simulink model "MSP_CurrentControl"  (R2018a)
settings: Solver=ode15s  StartTime=0.0  StopTime=1  RelTol=1e-3
values from neighbouring files (symbols this model uses):
  Kd = 0    [init.m]
  Ki = 63    [init.m]
  Kp = 6.3    [init.m]
  L = 1e-1    (= 0.1)    [init.m]
  n_levels = 9    [init.m]
  R = 90    [init.m]
  reference_frequency_hz = 100    [init.m]
  Ts = 1e-4    (= 0.0001)    [init.m]
  Vdc = 1    [init.m]
undefined symbols (not defined in the file or in its folder): G, serial
libraries: elec_lib x63, nesl_utility x52, powerlib x41, fl_lib x40, powerlib_meascontrol x4, simulink x3, instrumentlib x3
(part 1 of 2)
settings Model: Creator=Lewis  LastModifiedBy=Lewis
settings SolverCC: AutoInsertRateTranBlk=on  InsertRTBMode=Never (minimum delay)
settings SimscapeCC: SimscapeLogType=all

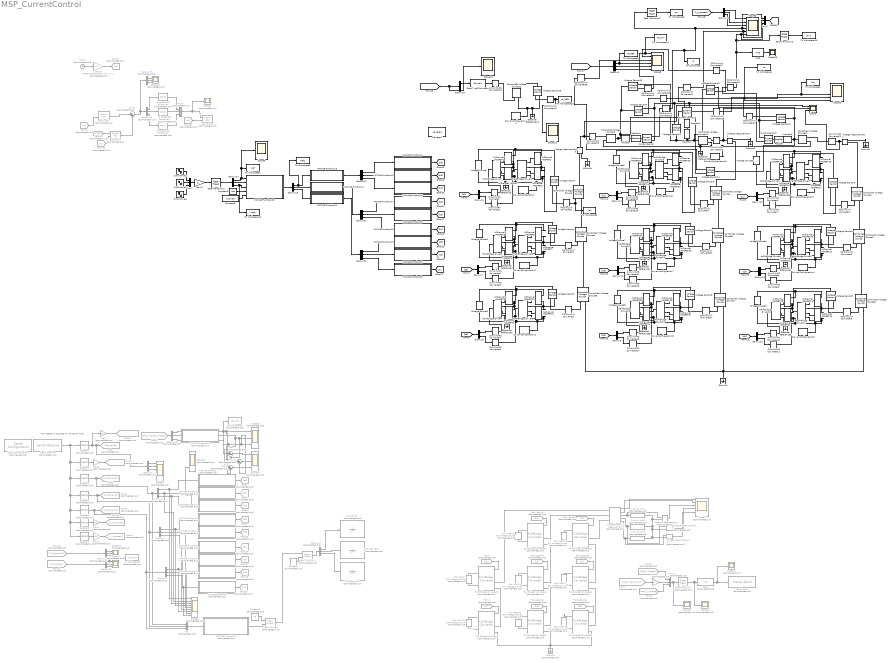
== system MSP_CurrentControl ==
  note: The header is dropped by the serial block
  1 ohm 5 mH1 : powerlib/Elements/Series RLC Branch  Commented=on  LConnTagsString=__new0  RConnTagsString=__new0  BranchType=RL  Resistance=R  Inductance=L  SetiL0=off  InitialCurrent=0  Capacitance=400e-6  Setx0=off  InitialVoltage=0  Measurements=None
  1 ohm 5 mH2 : powerlib/Elements/Series RLC Branch  Commented=on  LConnTagsString=__new0  RConnTagsString=__new0  BranchType=RL  Resistance=R  Inductance=L  SetiL0=off  InitialCurrent=0  Capacitance=400e-6  Setx0=off  InitialVoltage=0  Measurements=None
  1 ohm 5 mH3 : powerlib/Elements/Series RLC Branch  Commented=on  LConnTagsString=__new0  RConnTagsString=__new0  BranchType=RL  Resistance=R  Inductance=L  SetiL0=on  InitialCurrent=0  Capacitance=400e-6  Setx0=off  InitialVoltage=0  Measurements=None
  Cast : DataTypeConversion  Commented=on  OutDataTypeStr=int8  SaturateOnIntegerOverflow=on
  Clock1 : Clock  Commented=on
  Constant : Constant  Commented=on  Value=[9;3;1]
  Constant1 : Constant  Commented=on  Value=G
  Constant2 : Constant  Value=Vdc
  Constant3 : Constant  Value=n_levels
  Controlled Voltage Source{9..12} (4 alike) : fl_lib/Electrical/Electrical Sources/Controlled Voltage Source
  Controlled Voltage Source{,1..8} (9 alike) : powerlib/Electrical Sources/Controlled Voltage Source  Initialize=on  Source_Type=AC  Amplitude=0  Phase=0  Frequency=0  Measurements=None
  Current Sensor : fl_lib/Electrical/Electrical Sensors/Current Sensor
  Current Sensor1 : fl_lib/Electrical/Electrical Sensors/Current Sensor
  Current Sensor2 : fl_lib/Electrical/Electrical Sensors/Current Sensor
  Data Type Conversion : DataTypeConversion
  Demux{1..4,14..15,17..19,25} (10 alike) : Demux  Commented=on  Outputs=3
  Demux{6..13,16} (9 alike) : Demux  Outputs=2
  Demux{5,20..24,26..27} (8 alike) : Demux  Outputs=3
  Discrete PID Controller : simulink/Continuous/PID Controller  Commented=on  Controller=PID  TimeDomain=Discrete-time  SampleTime=-1  IntegratorMethod=Forward Euler  FilterMethod=Forward Euler  Form=Parallel  UseFilter=on  ControllerParametersSource=internal  P=Kp  I=Ki  D=Kd  N=100  InitialConditionSource=internal  InitialConditionForIntegrator=0  InitialConditionForFilter=0  ExternalReset=none  LimitOutput=off  UpperSaturationLimit=inf  LowerSaturationLimit=-inf  LinearizeAsGain=off  AntiWindupMode=none  Kb=1  TrackingMode=off  Kt=1  PParamMin=[]  PParamMax=[]  IParamMin=[]  IParamMax=[]  DParamMin=[]  DParamMax=[]  NParamMin=[]  NParamMax=[]  KbParamMin=[]  KbParamMax=[]  KtParamMin=[]  KtParamMax=[]  POutMin=[]  POutMax=[]  IOutMin=[]  IOutMax=[]  DOutMin=[]  DOutMax=[]  NOutMin=[]  NOutMax=[]  KbOutMin=[]  KbOutMax=[]  KtOutMin=[]  KtOutMax=[]  IntegratorOutMin=[]  IntegratorOutMax=[]  FilterOutMin=[]  FilterOutMax=[]  SumOutMin=[]  SumOutMax=[]  SumI1OutMin=[]  SumI1OutMax=[]  SumI2OutMin=[]  SumI2OutMax=[]  SumI3OutMin=[]  SumI3OutMax=[]  SumDOutMin=[]  SumDOutMax=[]  SaturationOutMin=[]  SaturationOutMax=[]  IntegratorContinuousStateAttributes=''  IntegratorStateMustResolveToSignalObject=off  IntegratorRTWStateStorageClass=Auto  FilterContinuousStateAttributes=''  FilterStateMustResolveToSignalObject=off  FilterRTWStateStorageClass=Auto  DifferentiatorICPrevScaledInput=0  DifferentiatorOutMin=[]  DifferentiatorOutMax=[]  FilterDiffOutCoefMin=[]  FilterDiffOutCoefMax=[]  SumDenOutMin=[]  SumDenOutMax=[]  SumNumOutMin=[]  SumNumOutMax=[]  ReciprocalOutMin=[]  ReciprocalOutMax=[]  DivideOutMin=[]  DivideOutMax=[]  TunerSelectOption=Transfer Function Based (PID Tuner App)
  Discrete PID Controller1 : simulink/Continuous/PID Controller  Commented=on  Controller=PID  TimeDomain=Discrete-time  SampleTime=-1  IntegratorMethod=Forward Euler  FilterMethod=Forward Euler  Form=Parallel  UseFilter=on  ControllerParametersSource=internal  P=Kp  I=Ki  D=Kd  N=100  InitialConditionSource=internal  InitialConditionForIntegrator=0  InitialConditionForFilter=0  ExternalReset=none  LimitOutput=off  UpperSaturationLimit=inf  LowerSaturationLimit=-inf  LinearizeAsGain=off  AntiWindupMode=none  Kb=1  TrackingMode=off  Kt=1  PParamMin=[]  PParamMax=[]  IParamMin=[]  IParamMax=[]  DParamMin=[]  DParamMax=[]  NParamMin=[]  NParamMax=[]  KbParamMin=[]  KbParamMax=[]  KtParamMin=[]  KtParamMax=[]  POutMin=[]  POutMax=[]  IOutMin=[]  IOutMax=[]  DOutMin=[]  DOutMax=[]  NOutMin=[]  NOutMax=[]  KbOutMin=[]  KbOutMax=[]  KtOutMin=[]  KtOutMax=[]  IntegratorOutMin=[]  IntegratorOutMax=[]  FilterOutMin=[]  FilterOutMax=[]  SumOutMin=[]  SumOutMax=[]  SumI1OutMin=[]  SumI1OutMax=[]  SumI2OutMin=[]  SumI2OutMax=[]  SumI3OutMin=[]  SumI3OutMax=[]  SumDOutMin=[]  SumDOutMax=[]  SaturationOutMin=[]  SaturationOutMax=[]  IntegratorContinuousStateAttributes=''  IntegratorStateMustResolveToSignalObject=off  IntegratorRTWStateStorageClass=Auto  FilterContinuousStateAttributes=''  FilterStateMustResolveToSignalObject=off  FilterRTWStateStorageClass=Auto  DifferentiatorICPrevScaledInput=0  DifferentiatorOutMin=[]  DifferentiatorOutMax=[]  FilterDiffOutCoefMin=[]  FilterDiffOutCoefMax=[]  SumDenOutMin=[]  SumDenOutMax=[]  SumNumOutMin=[]  SumNumOutMax=[]  ReciprocalOutMin=[]  ReciprocalOutMax=[]  DivideOutMin=[]  DivideOutMax=[]  TunerSelectOption=Transfer Function Based (PID Tuner App)
  Discrete PID Controller2 : simulink/Continuous/PID Controller  Commented=on  Controller=PID  TimeDomain=Discrete-time  SampleTime=-1  IntegratorMethod=Forward Euler  FilterMethod=Forward Euler  Form=Parallel  UseFilter=on  ControllerParametersSource=internal  P=Kp  I=Ki  D=Kd  N=100  InitialConditionSource=internal  InitialConditionForIntegrator=0  InitialConditionForFilter=0  ExternalReset=none  LimitOutput=off  UpperSaturationLimit=inf  LowerSaturationLimit=-inf  LinearizeAsGain=off  AntiWindupMode=none  Kb=1  TrackingMode=off  Kt=1  PParamMin=[]  PParamMax=[]  IParamMin=[]  IParamMax=[]  DParamMin=[]  DParamMax=[]  NParamMin=[]  NParamMax=[]  KbParamMin=[]  KbParamMax=[]  KtParamMin=[]  KtParamMax=[]  POutMin=[]  POutMax=[]  IOutMin=[]  IOutMax=[]  DOutMin=[]  DOutMax=[]  NOutMin=[]  NOutMax=[]  KbOutMin=[]  KbOutMax=[]  KtOutMin=[]  KtOutMax=[]  IntegratorOutMin=[]  IntegratorOutMax=[]  FilterOutMin=[]  FilterOutMax=[]  SumOutMin=[]  SumOutMax=[]  SumI1OutMin=[]  SumI1OutMax=[]  SumI2OutMin=[]  SumI2OutMax=[]  SumI3OutMin=[]  SumI3OutMax=[]  SumDOutMin=[]  SumDOutMax=[]  SaturationOutMin=[]  SaturationOutMax=[]  IntegratorContinuousStateAttributes=''  IntegratorStateMustResolveToSignalObject=off  IntegratorRTWStateStorageClass=Auto  FilterContinuousStateAttributes=''  FilterStateMustResolveToSignalObject=off  FilterRTWStateStorageClass=Auto  DifferentiatorICPrevScaledInput=0  DifferentiatorOutMin=[]  DifferentiatorOutMax=[]  FilterDiffOutCoefMin=[]  FilterDiffOutCoefMax=[]  SumDenOutMin=[]  SumDenOutMax=[]  SumNumOutMin=[]  SumNumOutMax=[]  ReciprocalOutMin=[]  ReciprocalOutMax=[]  DivideOutMin=[]  DivideOutMax=[]  TunerSelectOption=Transfer Function Based (PID Tuner App)
  Electrical Reference{,1..10} (11 alike) : fl_lib/Electrical/Electrical Elements/Electrical Reference
  From : From  Commented=on  GotoTag=a3
  From1 : From  Commented=on  GotoTag=a9
  From10 : From  Commented=on  GotoTag=V_XN_sensed
  From11 : From  Commented=on  GotoTag=I_ll_sensed
  From2 : From  Commented=on  GotoTag=abc_inverter_voltage
  From20 : From  Commented=on  GotoTag=I_meas
  From21 : From  Commented=on  GotoTag=wt
  From22 : From  Commented=on  GotoTag=wt
  From23 : From  Commented=on  GotoTag=wt
  From3 : From  Commented=on  GotoTag=load_voltage
  From4 : From  Commented=on  GotoTag=load_line_current
  From5 : From  Commented=on  GotoTag=load_ll_voltage
  From_Boost1 : From  Commented=on  GotoTag=b1
  From_Boost2 : From  Commented=on  GotoTag=c1
  From_Boost3 : From  Commented=on  GotoTag=c3
  From_Boost4 : From  Commented=on  GotoTag=c9
  From_Boost5 : From  Commented=on  GotoTag=b3
  From_Boost6 : From  Commented=on  GotoTag=b9
  Full-Bridge Converter : powerlib/Power Electronics/Full-Bridge Converter  Commented=on  ModelType=Switching devices  Ron=Ron  Rs=1e6  Cs=1e-3  Vforward=[ 0, 0 ]  Ron_Diode=1e-3  Rs_Diode=1e6  Cs_Diode=inf  Vf_Diode=1e-3  Rs_CurrentSource=1
      settings: AttributesFormatString=%<ModelType>  SourceProductName=Simscape Power Systems  SourceProductBaseCode=PS
  Full-Bridge Converter{1,4..8} (6 alike) : powerlib/Power Electronics/Full-Bridge Converter  Commented=on  ModelType=Switching devices  Ron=Ron  Rs=1e6  Cs=inf  Vforward=[ 0, 0 ]  Ron_Diode=1e-3  Rs_Diode=1e6  Cs_Diode=inf  Vf_Diode=1e-3  Rs_CurrentSource=1
      settings: AttributesFormatString=%<ModelType>  SourceProductName=Simscape Power Systems  SourceProductBaseCode=PS
  Full-Bridge Converter2 : powerlib/Power Electronics/Full-Bridge Converter  Commented=on  ModelType=Switching devices  Ron=Ron  Rs=1e6  Cs=1e-3  Vforward=[ 0, 0 ]  Ron_Diode=1e-3  Rs_Diode=1e6  Cs_Diode=inf  Vf_Diode=1e-3  Rs_CurrentSource=1
      settings: AttributesFormatString=%<ModelType>  SourceProductName=Simscape Power Systems  SourceProductBaseCode=PS
  Gain : Gain  Commented=on  Gain=Vdc
  Gain2 : Gain  Commented=on  Gain=64
  Gain3 : Gain  Commented=on  Gain=1/20
  Gain4 : Gain  Commented=on  Gain=1/2
  Gain5 : Gain  Gain=6
  Gain6 : Gain  Commented=on  Gain=reference_frequency_hz * 2 * pi
  Gain7 : Gain  Commented=on  Gain=1/64
  Goto : Goto  Commented=on  GotoTag=abc_levels
  Goto1 : Goto  Commented=on  GotoTag=ll_abc_reference
  Goto10 : Goto  Commented=on  GotoTag=V_XN_sensed
  Goto11 : Goto  Commented=on  GotoTag=I_ll_sensed
  Goto12 : Goto  Commented=on  GotoTag=b3
  Goto13 : Goto  Commented=on  GotoTag=b1
  Goto14 : Goto  Commented=on  GotoTag=c9
  Goto15 : Goto  Commented=on  GotoTag=c3
  Goto16 : Goto  Commented=on  GotoTag=c1
  Goto2 : Goto  Commented=on  GotoTag=a9
  Goto27 : Goto  Commented=on  GotoTag=wt
  Goto3 : Goto  Commented=on  GotoTag=a_cell_levels
  Goto4 : Goto  Commented=on  GotoTag=b_cell_levels
  Goto5 : Goto  Commented=on  GotoTag=c_cell_levels
  Goto6 : Goto  Commented=on  GotoTag=abc_inverter_voltage
  Goto7 : Goto  Commented=on  GotoTag=a3
  Goto8 : Goto  Commented=on  GotoTag=a1
  Goto9 : Goto  Commented=on  GotoTag=b9
  Ground : powerlib/Elements/Ground  Commented=on  LConnTagsString=a
  Ground{1..4} (4 alike) : powerlib/Elements/Ground  LConnTagsString=a
  Half-Bridge Driver{,1..17} (18 alike) : elec_lib/Actuators & Drivers/Drivers/Half-Bridge Driver  vHigh=15 V  vLow=0 V  parameterization=1  rHigh=2 Ohm  rLow=2 Ohm  tRise=20 ns  tFall=20 ns  cLoad=10 nF  enable_faults=0  t_fault=1 s  fault_type=1  uHighValue=0.7  uLowValue=0.3  tpLH=50 ns  tdLH=100 ns  tpHL=50 ns  tdHL=100 ns  ZonTime_specify=off  ZonTime_priority=None  ZonTime=0 s  ZoffTime_specify=off  ZoffTime_priority=None  ZoffTime=0 s  power_dissipated_high_side_specify=off  power_dissipated_high_side_priority=None  power_dissipated_high_side=0 W  power_dissipated_high_side_nominal_specify=off  power_dissipated_high_side_nominal_unit=W  power_dissipated_high_side_nominal_value=1  power_dissipated_low_side_specify=off  power_dissipated_low_side_priority=None  power_dissipated_low_side=0 W  power_dissipated_low_side_nominal_specify=off  power_dissipated_low_side_nominal_unit=W  power_dissipated_low_side_nominal_value=1  uHigh=2.0 V  uLow=0.8 V
      settings: SourceProductName=Simscape Electronics  SourceProductBaseCode=SN
  Inductor : fl_lib/Electrical/Electrical Elements/Inductor  l=L H  r=0 Ohm  g=1e-9 1/Ohm  i_specify=off  i_priority=None  i=0 A  i_nominal_specify=off  i_nominal_unit=A  i_nominal_value=1  v_specify=off  v_priority=None  v=0 V  v_nominal_specify=off  v_nominal_unit=V  v_nominal_value=1  i_L_specify=off  i_L_priority=High  i_L=0 A  i_L_nominal_specify=off  i_L_nominal_unit=A  i_L_nominal_value=1
  Inductor1 : fl_lib/Electrical/Electrical Elements/Inductor  l=L H  r=0 Ohm  g=1e-9 1/Ohm  i_specify=off  i_priority=None  i=0 A  i_nominal_specify=off  i_nominal_unit=A  i_nominal_value=1  v_specify=off  v_priority=None  v=0 V  v_nominal_specify=off  v_nominal_unit=V  v_nominal_value=1  i_L_specify=off  i_L_priority=High  i_L=0 A  i_L_nominal_specify=off  i_L_nominal_unit=A  i_L_nominal_value=1
  Inductor2 : fl_lib/Electrical/Electrical Elements/Inductor  l=L H  r=0 Ohm  g=1e-9 1/Ohm  i_specify=off  i_priority=None  i=0 A  i_nominal_specify=off  i_nominal_unit=A  i_nominal_value=1  v_specify=off  v_priority=None  v=0 V  v_nominal_specify=off  v_nominal_unit=V  v_nominal_value=1  i_L_specify=off  i_L_priority=High  i_L=0 A  i_L_nominal_specify=off  i_L_nominal_unit=A  i_L_nominal_value=1
  MATLAB Function : MATLAB Function  Commented=on  TreatAsAtomicUnit=on
  MATLAB Function1 : MATLAB Function  Commented=on  TreatAsAtomicUnit=on
  MATLAB Function10 : MATLAB Function  Commented=on  TreatAsAtomicUnit=on
  MATLAB Function11 : MATLAB Function  TreatAsAtomicUnit=on
  MATLAB Function12 : MATLAB Function  TreatAsAtomicUnit=on
  MATLAB Function13 : MATLAB Function  TreatAsAtomicUnit=on
  MATLAB Function14 : MATLAB Function  TreatAsAtomicUnit=on
  MATLAB Function15 : MATLAB Function  TreatAsAtomicUnit=on
  MATLAB Function16 : MATLAB Function  TreatAsAtomicUnit=on
  MATLAB Function17 : MATLAB Function  TreatAsAtomicUnit=on
  MATLAB Function18 : MATLAB Function  TreatAsAtomicUnit=on
  MATLAB Function19 : MATLAB Function  TreatAsAtomicUnit=on
  MATLAB Function2 : MATLAB Function  Commented=on  TreatAsAtomicUnit=on
  MATLAB Function20 : MATLAB Function  TreatAsAtomicUnit=on
  MATLAB Function21 : MATLAB Function  TreatAsAtomicUnit=on
  MATLAB Function22 : MATLAB Function  TreatAsAtomicUnit=on
  MATLAB Function23 : MATLAB Function  TreatAsAtomicUnit=on
  MATLAB Function24 : MATLAB Function  Commented=on  TreatAsAtomicUnit=on
  MATLAB Function3 : MATLAB Function  Commented=on  TreatAsAtomicUnit=on
  MATLAB Function4 : MATLAB Function  Commented=on  TreatAsAtomicUnit=on
  MATLAB Function5 : MATLAB Function  Commented=on  TreatAsAtomicUnit=on
  MATLAB Function6 : MATLAB Function  Commented=on  TreatAsAtomicUnit=on
  MATLAB Function7 : MATLAB Function  Commented=on  TreatAsAtomicUnit=on
  MATLAB Function8 : MATLAB Function  Commented=on  TreatAsAtomicUnit=on
  Matrix Multiply : Product  Commented=on  Multiplication=Matrix(*)
  Matrix Multiply1 : Product  Commented=on  Multiplication=Matrix(*)
  Mux : Mux  Commented=on  Inputs=3
  Mux1 : Mux  Inputs=3
  Mux2 : Mux  Inputs=3
  Mux3 : Mux  Commented=on  Inputs=3
  Mux4 : Mux  Commented=on  Inputs=3
  N-Channel MOSFET{,4,8,12,18,22,24,30,34} (9 alike) : elec_lib/Semiconductor Devices/N-Channel MOSFET  parameterization=1  prmDatasheet=1  prmEquCoeff=1  Beta=5 A/V^2  Rds=0.025 Ohm  Id=6 A  Vgs=10 V  Vth=1.7 V  lam=0 1/V  Tmeas=25 degC  RS=1e-4 Ohm  RD=0.01 Ohm  C_param=3  C_GS=270 pF  C_GD=80 pF  C_DS=0 pF  C_iss=350 pF  C_rss=80 pF  C_oss=0 pF  C_GS_vec=[ 270 300 290 280 295 255 ] pF  C_GD_vec=[ 450 400 300 190 95 55 ] pF  C_DS_vec=[ 450 410 390 230 175 115 ] pF  C_iss_vec=[ 720 700 590 470 390 310 ] pF  C_rss_vec=[ 450 400 300 190 95 55 ] pF  C_oss_vec=[ 900 810 690 420 270 170 ] pF  C_Vds_vec=[ 0.1 0.3 1 3 10 30 ] V  V_GS_for_cap_data=0 V  charge_linearity_param=1  C_OX=200 pF  V_C_OX=-0.5 V  IsDiode=0 A  Vbi=0.6 V  n=1  Cj0Diode=0 pF  TT=50e-9 s  dVth_dT=-6 mV/K  Rds_T2=0.037 Ohm  Tmeas2=125 degC  BEXDatasheet=-1.5  BEXEquCoeff=-1.5  etaisDatasheet=3  etaisEquCoeff=3  TdeviceDatasheet=25 degC  TdeviceEquCoeff=25 degC  Rth=[1, 10] K/W  thermal_mass_parameterization=1  thermal_mass=[1, 1] J/K  thermal_time_constant=[1, 10] s  thermal_mass_initial_temperatures=[ 25 25 ] degC  betaref=18 A/V^2  Vfbref=-1.1 V  gamma=3.5 V^0.50000  phib2ref=1 V  thesatref=0.4 1/V  alpha=0  Vp=5e-2 V  thesrref=0 1/V  m=8  Tref=25 degC  Cox=1500 pF  Cgso=100 pF  Cgdo=14 pF  Rsref=2e-3 Ohm  Rdref=0.17 Ohm  Rgref=8.4 Ohm  Isref=5.2e-13 A  Cj0=480 pF  Tprm=1  etabet=1.3  Stvfb=5e-4 V/K  Stphib=-8.5e-4 V/K  etasat=1.04  etasr=0.65  etar=0.95  etais=3  Tsim=25 degC  T0=[25, 25] degC
      settings: SourceProductName=Simscape Electronics  SourceProductBaseCode=SN
  N-Channel MOSFET{1..3,5..7,9..11,13..17,19..21,23,26..29,31..33,35} (26 alike) : elec_lib/Semiconductor Devices/N-Channel MOSFET  parameterization=1  prmDatasheet=1  prmEquCoeff=1  Beta=5 A/V^2  Rds=0.025 Ohm  Id=6 A  Vgs=10 V  Vth=1.7 V  lam=0 1/V  Tmeas=25 degC  RS=1e-4 Ohm  RD=0.01 Ohm  C_param=1  C_GS=270 pF  C_GD=80 pF  C_DS=0 pF  C_iss=350 pF  C_rss=80 pF  C_oss=0 pF  C_GS_vec=[ 270 300 290 280 295 255 ] pF  C_GD_vec=[ 450 400 300 190 95 55 ] pF  C_DS_vec=[ 450 410 390 230 175 115 ] pF  C_iss_vec=[ 720 700 590 470 390 310 ] pF  C_rss_vec=[ 450 400 300 190 95 55 ] pF  C_oss_vec=[ 900 810 690 420 270 170 ] pF  C_Vds_vec=[ 0.1 0.3 1 3 10 30 ] V  V_GS_for_cap_data=0 V  charge_linearity_param=1  C_OX=200 pF  V_C_OX=-0.5 V  IsDiode=0 A  Vbi=0.6 V  n=1  Cj0Diode=0 pF  TT=50e-9 s  dVth_dT=-6 mV/K  Rds_T2=0.037 Ohm  Tmeas2=125 degC  BEXDatasheet=-1.5  BEXEquCoeff=-1.5  etaisDatasheet=3  etaisEquCoeff=3  TdeviceDatasheet=25 degC  TdeviceEquCoeff=25 degC  Rth=[1, 10] K/W  thermal_mass_parameterization=1  thermal_mass=[1, 1] J/K  thermal_time_constant=[1, 10] s  thermal_mass_initial_temperatures=[ 25 25 ] degC  betaref=18 A/V^2  Vfbref=-1.1 V  gamma=3.5 V^0.50000  phib2ref=1 V  thesatref=0.4 1/V  alpha=0  Vp=5e-2 V  thesrref=0 1/V  m=8  Tref=25 degC  Cox=1500 pF  Cgso=100 pF  Cgdo=14 pF  Rsref=2e-3 Ohm  Rdref=0.17 Ohm  Rgref=8.4 Ohm  Isref=5.2e-13 A  Cj0=480 pF  Tprm=1  etabet=1.3  Stvfb=5e-4 V/K  Stphib=-8.5e-4 V/K  etasat=1.04  etasr=0.65  etar=0.95  etais=3  Tsim=25 degC  T0=[25, 25] degC
      settings: SourceProductName=Simscape Electronics  SourceProductBaseCode=SN
  N-Channel MOSFET25 : elec_lib/Semiconductor Devices/N-Channel MOSFET  parameterization=1  prmDatasheet=1  prmEquCoeff=1  Beta=5 A/V^2  Rds=0.025 Ohm  Id=6 A  Vgs=10 V  Vth=1.7 V  lam=0 1/V  Tmeas=25 degC  RS=1e-4 Ohm  RD=0.01 Ohm  C_param=2  C_GS=270 pF  C_GD=80 pF  C_DS=0 pF  C_iss=350 pF  C_rss=80 pF  C_oss=0 pF  C_GS_vec=[ 270 300 290 280 295 255 ] pF  C_GD_vec=[ 450 400 300 190 95 55 ] pF  C_DS_vec=[ 450 410 390 230 175 115 ] pF  C_iss_vec=[ 720 700 590 470 390 310 ] pF  C_rss_vec=[ 450 400 300 190 95 55 ] pF  C_oss_vec=[ 900 810 690 420 270 170 ] pF  C_Vds_vec=[ 0.1 0.3 1 3 10 30 ] V  V_GS_for_cap_data=0 V  charge_linearity_param=1  C_OX=200 pF  V_C_OX=-0.5 V  IsDiode=0 A  Vbi=0.6 V  n=1  Cj0Diode=0 pF  TT=50e-9 s  dVth_dT=-6 mV/K  Rds_T2=0.037 Ohm  Tmeas2=125 degC  BEXDatasheet=-1.5  BEXEquCoeff=-1.5  etaisDatasheet=3  etaisEquCoeff=3  TdeviceDatasheet=25 degC  TdeviceEquCoeff=25 degC  Rth=[1, 10] K/W  thermal_mass_parameterization=1  thermal_mass=[1, 1] J/K  thermal_time_constant=[1, 10] s  thermal_mass_initial_temperatures=[ 25 25 ] degC  betaref=18 A/V^2  Vfbref=-1.1 V  gamma=3.5 V^0.50000  phib2ref=1 V  thesatref=0.4 1/V  alpha=0  Vp=5e-2 V  thesrref=0 1/V  m=8  Tref=25 degC  Cox=1500 pF  Cgso=100 pF  Cgdo=14 pF  Rsref=2e-3 Ohm  Rdref=0.17 Ohm  Rgref=8.4 Ohm  Isref=5.2e-13 A  Cj0=480 pF  Tprm=1  etabet=1.3  Stvfb=5e-4 V/K  Stphib=-8.5e-4 V/K  etasat=1.04  etasr=0.65  etar=0.95  etais=3  Tsim=25 degC  T0=[25, 25] degC
      settings: SourceProductName=Simscape Electronics  SourceProductBaseCode=SN
  PS-Simulink Converter{1..19} (19 alike) : nesl_utility/PS-Simulink Converter  PhysicalDomain=network_engine_domain  SubClassName=ps_output  LeftPortType=input  RightPortType=output  PseudoPeriodic=off  Frequencies=[]  Unit=1  AffineConversion=off
  Rate Transition : RateTransition  Commented=on  OutPortSampleTime=Ts
  Rate Transition1 : RateTransition  OutPortSampleTime=Ts
  Rate Transition2 : RateTransition  OutPortSampleTime=Ts
  Rate Transition3 : RateTransition  OutPortSampleTime=Ts
  Resistor : fl_lib/Electrical/Electrical Elements/Resistor  R=R Ohm  i_specify=off  i_priority=None  i=0 A  i_nominal_specify=off  i_nominal_unit=A  i_nominal_value=1  v_specify=off  v_priority=None  v=0 V  v_nominal_specify=off  v_nominal_unit=V  v_nominal_value=1
  Resistor1 : fl_lib/Electrical/Electrical Elements/Resistor  R=R Ohm  i_specify=off  i_priority=None  i=0 A  i_nominal_specify=off  i_nominal_unit=A  i_nominal_value=1  v_specify=off  v_priority=None  v=0 V  v_nominal_specify=off  v_nominal_unit=V  v_nominal_value=1
  Resistor2 : fl_lib/Electrical/Electrical Elements/Resistor  R=R Ohm  i_specify=off  i_priority=None  i=0 A  i_nominal_specify=off  i_nominal_unit=A  i_nominal_value=1  v_specify=off  v_priority=None  v=0 V  v_nominal_specify=off  v_nominal_unit=V  v_nominal_value=1
  Scope : Scope  NumInputPorts=3
  Scope1 : Scope  Commented=on  NumInputPorts=9
  Scope{7,10..12} (4 alike) : Scope  Commented=on
  Scope{6,13,18..19} (4 alike) : Scope
  Scope{8,14..17,20} (6 alike) : Scope  Commented=on  NumInputPorts=3
  Scope2 : Scope  Commented=on  NumInputPorts=6
  Scope3 : Scope  NumInputPorts=6
  Scope4 : Scope  Commented=on  NumInputPorts=6
  Scope5 : Scope  NumInputPorts=6
  Scope9 : Scope  NumInputPorts=6
  Selector : Selector  Commented=on  IndexMode=Zero-based  InputPortWidth=23  IndexOptions=Index vector (dialog)  Indices=[0:2]  OutputSizes=1
  Selector1 : Selector  Commented=on  IndexMode=Zero-based  InputPortWidth=23  IndexOptions=Index vector (dialog)  Indices=3:5  OutputSizes=1
  Selector2 : Selector  Commented=on  IndexMode=Zero-based  InputPortWidth=23  IndexOptions=Index vector (dialog)  Indices=6:8  OutputSizes=1
  Selector3 : Selector  Commented=on  IndexMode=Zero-based  InputPortWidth=23  IndexOptions=Index vector (dialog)  Indices=9:11  OutputSizes=1
  Selector4 : Selector  Commented=on  IndexMode=Zero-based  InputPortWidth=23  IndexOptions=Index vector (dialog)  Indices=12:14  OutputSizes=1
  Selector5 : Selector  Commented=on  IndexMode=Zero-based  InputPortWidth=23  IndexOptions=Index vector (dialog)  Indices=15:17  OutputSizes=1
  Selector6 : Selector  Commented=on  IndexMode=Zero-based  InputPortWidth=23  IndexOptions=Index vector (dialog)  Indices=18:20  OutputSizes=1
  Serial Configuration : instrumentlib/Serial Configuration  Priority=-200000  Commented=on  ComPortMenu=<Please select a port...>  ComPort=COM8  ObjConstructor=serial('COM8');  BaudRate=921600  DataBits=8  Parity=none  StopBits=1  FlowControl=none  Timeout=30  ByteOrder=LittleEndian
  Serial Receive : instrumentlib/Serial Receive  Commented=on  ComPortMenu=<Please select a port...>  ComPort=COM8  ObjConstructor=serial('COM8');  Header=Aa  Terminator=<none>  DataSize="[23   1]"  DataType=int8  EnableBlockingMode=on  ActionDataUnavailable=Output last received value  CustomValue=zeros(23,1)  SampleTime=Ts
  Serial Send : instrumentlib/Serial Send  Commented=on  ComPortMenu=<Please select a port...>  ComPort=COM8  ObjConstructor=serial('COM16');  Header=Aa  Terminator=<none>  EnableBlockingMode=on
  Simulink-PS Converter{,1..21} (22 alike) : nesl_utility/Simulink-PS Converter  PhysicalDomain=network_engine_domain  SubClassName=ps_input  LeftPortType=input  RightPortType=output  PseudoPeriodic=off  Frequencies=[]  NoiseDistribution=none  NoiseParameters=[]  Unit=1  AffineConversion=off  FilteringAndDerivatives=provide  SimscapeFilterOrder=1  InputFilterTimeConstant=0.001  UdotUserProvided=0
  Sine Wave1 : Sin  Frequency=reference_frequency_hz * 2 * pi  Samples=100  SampleTime=Ts
  Sine Wave2 : Sin  Frequency=reference_frequency_hz * 2 * pi  Phase=-2*pi/3  Samples=100  SampleTime=Ts  Offset=66
  Sine Wave6 : Sin  Frequency=reference_frequency_hz * 2 * pi  Phase=2*pi/3  Samples=100  SampleTime=Ts  Offset=33
  Solver Configuration{,1..10} (11 alike) : nesl_utility/Solver Configuration  PhysicalDomain=network_engine_domain  SubClassName=solver  LeftPortType=input  RightPortType=generic  Tones=[]  Harmonics=[]  SimulateNoise=off  Profile=off  UseLocalSampling=off  EnableSwitchedLinearOptims=on  FrequencyDomain=off  UseCCode=off  RelTol=0.001  AbsTol=1e-06  MinStep=1e-09  ToWorkspace=off  RevertToSquareIcSolve=off  NumHomotopyIterations=100  PhasorMode=off  PhasorModeNumHarmonics=1  DoDC=off  ResidualTolerance=1e-09  UseLocalSolver=off  LocalSolverChoice=NE_BACKWARD_EULER_ADVANCER  LocalSolverSampleTime=0.001  DoFixedCost=off  MaxNonlinIter=3  MaxModeIter=2  LinearAlgebra=Sparse  EquationFormulation=NE_TIME_EF  DelaysMemoryBudget=1024  AutomaticFiltering=on  FilteringTimeConstant=0.001
  Sum{,1..3} (4 alike) : Sum  Commented=on  Inputs=|+-
  THD : powerlib_meascontrol/Measurements/THD  Freq=100  Ts=0
  Three-Phase V-I Measurement : powerlib/Measurements/Three-Phase V-I Measurement  Commented=on  VoltageMeasurement=phase-to-ground  SetLabelV=off  LabelV=Vabc  Vpu=off  VpuLL=off  CurrentMeasurement=yes  SetLabelI=off  LabelI=Iabc  Ipu=off  Pbase=100e6  Vbase=500e3  OutputType=Complex  PhasorSimulation=off  PSBequivalent=0
  To Workspace : ToWorkspace  VariableName=Ia  SaveFormat=Timeseries  SampleTime=-1
  To Workspace1 : ToWorkspace  VariableName=Vref  SaveFormat=Timeseries  SampleTime=-1
  To Workspace10 : ToWorkspace  VariableName=Va_REF1  SaveFormat=Timeseries  SampleTime=-1
  To Workspace11 : ToWorkspace  VariableName=Va_Sim  SaveFormat=Timeseries  SampleTime=-1
  To Workspace12 : ToWorkspace  VariableName=Vrefc  SaveFormat=Timeseries  SampleTime=-1
  To Workspace13 : ToWorkspace  VariableName=Ian1  SaveFormat=Timeseries  SampleTime=-1
  To Workspace2 : ToWorkspace  VariableName=Va  SaveFormat=Timeseries  SampleTime=-1
  To Workspace3 : ToWorkspace  VariableName=Vref1  SaveFormat=Timeseries  SampleTime=-1
  To Workspace4 : ToWorkspace  VariableName=Van  SaveFormat=Timeseries  SampleTime=-1
  To Workspace5 : ToWorkspace  VariableName=Va1  SaveFormat=Timeseries  SampleTime=-1
  To Workspace6 : ToWorkspace  VariableName=Ian  SaveFormat=Timeseries  SampleTime=-1
  To Workspace7 : ToWorkspace  Commented=on  VariableName=Van_HW  SaveFormat=Timeseries  SampleTime=-1
  To Workspace8 : ToWorkspace  Commented=on  VariableName=Ian_HW1  SaveFormat=Timeseries  SampleTime=-1
  To Workspace9 : ToWorkspace  VariableName=Va_REF  SaveFormat=Timeseries  SampleTime=-1
  Transfer Fcn : TransferFcn  Commented=on  Denominator=[L R]
  Transfer Fcn1 : TransferFcn  Commented=on  Denominator=[L R]
  Transfer Fcn2 : TransferFcn  Commented=on  Denominator=[L R]
  Vdc/ (400V) : powerlib/Electrical Sources/DC Voltage Source  Commented=on  Amplitude=3  Measurements=None
  Vdc/ (400V)2 : powerlib/Electrical Sources/DC Voltage Source  Commented=on  Amplitude=9  Measurements=None
  Vdc/ (400V)3 : powerlib/Electrical Sources/DC Voltage Source  Commented=on  Amplitude=9  Measurements=None
  Vdc/ (400V)4 : powerlib/Electrical Sources/DC Voltage Source  Commented=on  Amplitude=3  Measurements=None
  Vdc/ (400V)5 : powerlib/Electrical Sources/DC Voltage Source  Commented=on  Amplitude=1  Measurements=None
  Vdc/ (400V)6 : powerlib/Electrical Sources/DC Voltage Source  Commented=on  Amplitude=1  Measurements=None
  Vdc/ (400V)7 : powerlib/Electrical Sources/DC Voltage Source  Commented=on  Amplitude=3  Measurements=None
  Vdc/ (400V)8 : powerlib/Electrical Sources/DC Voltage Source  Commented=on  Amplitude=9  Measurements=None
  Voltage Measurement : powerlib/Measurements/Voltage Measurement  Commented=on  PhasorSimulation=off  OutputType=Complex  PSBequivalent=0
  Voltage Measurement1 : powerlib/Measurements/Voltage Measurement  PhasorSimulation=off  OutputType=Complex  PSBequivalent=0
  Voltage Measurement2 : powerlib/Measurements/Voltage Measurement  Commented=on  PhasorSimulation=off  OutputType=Complex  PSBequivalent=0
  Voltage Measurement3 : powerlib/Measurements/Voltage Measurement  Commented=on  PhasorSimulation=off  OutputType=Complex  PSBequivalent=0
  Voltage Measurement4 : powerlib/Measurements/Voltage Measurement  PhasorSimulation=off  OutputType=Complex  PSBequivalent=0
  Voltage Measurement5 : powerlib/Measurements/Voltage Measurement  PhasorSimulation=off  OutputType=Complex  PSBequivalent=0
  Voltage Sensor{,1..15} (16 alike) : fl_lib/Electrical/Electrical Sensors/Voltage Sensor
  Voltage Source : elec_lib/Sources/Voltage Source  dc_voltage=1 V  ac_voltage=0 V  ac_shift=0 rad  ac_frequency=60 Hz  noise_mode=0  PSD=0 V^2/Hz  repeatability=1  auto_seed=1254062075  user_seed=0  sample_time=1e-3 s  i_specify=off  i_priority=None  i=0 A  i_nominal_specify=off  i_nominal_unit=A  i_nominal_value=1  v_specify=off  v_priority=None  v=0 V  v_nominal_specify=off  v_nominal_unit=V  v_nominal_value=1
      settings: SourceProductName=Simscape Electronics  SourceProductBaseCode=SN
  Voltage Source1 : elec_lib/Sources/Voltage Source  dc_voltage=3 V  ac_voltage=0 V  ac_shift=0 rad  ac_frequency=60 Hz  noise_mode=0  PSD=0 V^2/Hz  repeatability=1  auto_seed=1234490714  user_seed=0  sample_time=1e-3 s  i_specify=off  i_priority=None  i=0 A  i_nominal_specify=off  i_nominal_unit=A  i_nominal_value=1  v_specify=off  v_priority=None  v=0 V  v_nominal_specify=off  v_nominal_unit=V  v_nominal_value=1
      settings: SourceProductName=Simscape Electronics  SourceProductBaseCode=SN
  Voltage Source2 : elec_lib/Sources/Voltage Source  dc_voltage=9 V  ac_voltage=0 V  ac_shift=0 rad  ac_frequency=60 Hz  noise_mode=0  PSD=0 V^2/Hz  repeatability=1  auto_seed=3890346746  user_seed=0  sample_time=1e-3 s  i_specify=off  i_priority=None  i=0 A  i_nominal_specify=off  i_nominal_unit=A  i_nominal_value=1  v_specify=off  v_priority=None  v=0 V  v_nominal_specify=off  v_nominal_unit=V  v_nominal_value=1
      settings: SourceProductName=Simscape Electronics  SourceProductBaseCode=SN
  Voltage Source3 : elec_lib/Sources/Voltage Source  dc_voltage=1 V  ac_voltage=0 V  ac_shift=0 rad  ac_frequency=60 Hz  noise_mode=0  PSD=0 V^2/Hz  repeatability=1  auto_seed=609397185  user_seed=0  sample_time=1e-3 s  i_specify=off  i_priority=None  i=0 A  i_nominal_specify=off  i_nominal_unit=A  i_nominal_value=1  v_specify=off  v_priority=None  v=0 V  v_nominal_specify=off  v_nominal_unit=V  v_nominal_value=1
      settings: SourceProductName=Simscape Electronics  SourceProductBaseCode=SN
  Voltage Source4 : elec_lib/Sources/Voltage Source  dc_voltage=3 V  ac_voltage=0 V  ac_shift=0 rad  ac_frequency=60 Hz  noise_mode=0  PSD=0 V^2/Hz  repeatability=1  auto_seed=1811450916  user_seed=0  sample_time=1e-3 s  i_specify=off  i_priority=None  i=0 A  i_nominal_specify=off  i_nominal_unit=A  i_nominal_value=1  v_specify=off  v_priority=None  v=0 V  v_nominal_specify=off  v_nominal_unit=V  v_nominal_value=1
      settings: SourceProductName=Simscape Electronics  SourceProductBaseCode=SN
  Voltage Source5 : elec_lib/Sources/Voltage Source  dc_voltage=9 V  ac_voltage=0 V  ac_shift=0 rad  ac_frequency=60 Hz  noise_mode=0  PSD=0 V^2/Hz  repeatability=1  auto_seed=3933054132  user_seed=0  sample_time=1e-3 s  i_specify=off  i_priority=None  i=0 A  i_nominal_specify=off  i_nominal_unit=A  i_nominal_value=1  v_specify=off  v_priority=None  v=0 V  v_nominal_specify=off  v_nominal_unit=V  v_nominal_value=1
      settings: SourceProductName=Simscape Electronics  SourceProductBaseCode=SN
  Voltage Source6 : elec_lib/Sources/Voltage Source  dc_voltage=1 V  ac_voltage=0 V  ac_shift=0 rad  ac_frequency=60 Hz  noise_mode=0  PSD=0 V^2/Hz  repeatability=1  auto_seed=4111000739  user_seed=0  sample_time=1e-3 s  i_specify=off  i_priority=None  i=0 A  i_nominal_specify=off  i_nominal_unit=A  i_nominal_value=1  v_specify=off  v_priority=None  v=0 V  v_nominal_specify=off  v_nominal_unit=V  v_nominal_value=1
      settings: SourceProductName=Simscape Electronics  SourceProductBaseCode=SN
  Voltage Source7 : elec_lib/Sources/Voltage Source  dc_voltage=3 V  ac_voltage=0 V  ac_shift=0 rad  ac_frequency=60 Hz  noise_mode=0  PSD=0 V^2/Hz  repeatability=1  auto_seed=2084672538  user_seed=0  sample_time=1e-3 s  i_specify=off  i_priority=None  i=0 A  i_nominal_specify=off  i_nominal_unit=A  i_nominal_value=1  v_specify=off  v_priority=None  v=0 V  v_nominal_specify=off  v_nominal_unit=V  v_nominal_value=1
      settings: SourceProductName=Simscape Electronics  SourceProductBaseCode=SN
  Voltage Source8 : elec_lib/Sources/Voltage Source  dc_voltage=9 V  ac_voltage=0 V  ac_shift=0 rad  ac_frequency=60 Hz  noise_mode=0  PSD=0 V^2/Hz  repeatability=1  auto_seed=3437178441  user_seed=0  sample_time=1e-3 s  i_specify=off  i_priority=None  i=0 A  i_nominal_specify=off  i_nominal_unit=A  i_nominal_value=1  v_specify=off  v_priority=None  v=0 V  v_nominal_specify=off  v_nominal_unit=V  v_nominal_value=1
      settings: SourceProductName=Simscape Electronics  SourceProductBaseCode=SN
  abc to dq0 : powerlib_meascontrol/Transformations/abc to dq0  Commented=on  Alignment=90 degrees behind phase A axis
  abc to dq1 : powerlib_meascontrol/Transformations/abc to dq0  Commented=on  Alignment=90 degrees behind phase A axis
  dq0 to abc1 : powerlib_meascontrol/Transformations/dq0 to abc  Commented=on  Alignment=90 degrees behind phase A axis
  powergui : powerlib/powergui  Priority=1  SimulationMode=Continuous  SampleTime=Ts  frequency=60  Iterations=50  frequencyindice=0  Pbase=100e6  ErrMax=1e-4  UnitsV=kV  UnitsW=MW  buscounter=0  FunctionMessages=off  echomessages=off  EnableUseOfTLC=off  CurrentSourceSwitches=off  DisableSnubberDevices=off  DisableRonSwitches=off  DisableVfSwitches=off  DisplayEquations=off  SolverType=Tustin/Backward Euler (TBE)  Interpol=off  ExternalGateDelay=off  methode=off  Ts=100  x0status=blocks  SPID=off  SwTol=0  HookPort=off  RestoreLinks=warning  ResistiveCurrentMeasurement=off  Frange=[0:2:500]  Ylog=off  Xlog=on  ShowGrid=off  save=off  variable=ZData  structure=0  ZoomFFT=off  StartTime=0.0  cycles=1  DisplayStyle=1  fundamental=60  FreqAxis=off  MaxFrequency=1000  frequencyindicesteady=1  RmsSteady=1  display=off
  wires:
  Demux4/3 -> Scope4/3
  Serial Receive/1 -> Selector3/1, Selector6/1, Selector5/1, Selector4/1, Selector2/1, Selector1/1, Selector/1
  Gain7/1 -> Goto11/1
  Gain4/1 -> Goto10/1
  Demux14/3 -> Scope15/3  "Vcn"
  Gain/1 -> Goto6/1
  Demux14/2 -> Scope15/2  "Vbn"
  From10/1 -> Demux14/1
  Demux1/1 -> Scope1/1, MATLAB Function/1(u)  "a9"
  Demux1/3 -> Scope17/3, MATLAB Function2/1(u), Scope1/3  "a1"
  Demux3/1 -> MATLAB Function6/1(u), Scope1/7  "c9"
  Demux1/2 -> MATLAB Function1/1(u), Scope1/2  "a3"
  Demux4/2 -> Scope4/2
  Selector3/1 -> Mux/2, Demux2/1, Goto4/1
  Demux2/1 -> MATLAB Function3/1(u), Scope1/4  "b9"
  Demux4/1 -> Scope4/1
  Demux14/1 -> Scope15/1  "Van"
  Selector5/1 -> Gain4/1
  Selector2/1 -> Mux/1, Demux1/1, Goto3/1  "a_cell_levels"
  Selector4/1 -> Mux/3, Demux3/1, Goto5/1
  Selector1/1 -> Gain3/1
  Demux3/2 -> MATLAB Function7/1(u), Scope1/8  "c3"
  Demux3/3 -> MATLAB Function8/1(u), Scope1/9  "c1"
  Selector6/1 -> Gain7/1
  Selector/1 -> Gain/1, Demux4/1, Goto/1
  Demux2/2 -> MATLAB Function4/1(u), Scope1/5  "b3"
  Demux15/3 -> Scope16/3  "ICc"
  Demux15/2 -> Scope16/2  "IBb"
  Demux15/1 -> To Workspace8/1, Scope16/1  "IAa"
  From11/1 -> Demux15/1
  Demux2/3 -> MATLAB Function5/1(u), Scope1/6  "b1"
  MATLAB Function/1(y) -> Goto2/1
  From_Boost1/1 -> Full-Bridge Converter4/1
  From_Boost2/1 -> Full-Bridge Converter5/1
  From_Boost3/1 -> Full-Bridge Converter1/1
  MATLAB Function1/1(y) -> Goto7/1
  MATLAB Function2/1(y) -> Goto8/1
  MATLAB Function8/1(y) -> Goto16/1
  MATLAB Function7/1(y) -> Goto15/1
  MATLAB Function6/1(y) -> Goto14/1
  MATLAB Function5/1(y) -> Goto13/1
  MATLAB Function4/1(y) -> Goto12/1
  MATLAB Function3/1(y) -> Goto9/1
  From_Boost4/1 -> Full-Bridge Converter8/1
  From_Boost5/1 -> Full-Bridge Converter6/1
  From_Boost6/1 -> Full-Bridge Converter7/1
  From/1 -> Full-Bridge Converter2/1
  From1/1 -> Full-Bridge Converter/1
  Three-Phase V-I Measurement/1 -> Scope2/1
  Three-Phase V-I Measurement/2 -> Scope2/2
  From3/1 -> Mux3/1
  Mux3/1 -> Scope11/1, Rate Transition/1
  From4/1 -> Gain2/1
  Rate Transition/1 -> Scope12/1, Cast/1
  From5/1 -> Mux3/3
  Cast/1 -> Scope10/1, Serial Send/1
  Gain2/1 -> Mux3/2
  Voltage Measurement/1 -> Scope2/3
  Voltage Measurement2/1 -> Scope2/4
  Voltage Measurement3/1 -> Scope2/5
  [a1] -> Demux6/1
  Demux17/3 -> Transfer Fcn2/1
  Demux17/2 -> Transfer Fcn1/1
  Demux17/1 -> Transfer Fcn/1
  Demux6/1 -> Simulink-PS Converter/1
  [a3] -> Demux7/1
  Demux7/1 -> Simulink-PS Converter2/1
  Demux7/2 -> Simulink-PS Converter3/1
  PS-Simulink Converter1/1 -> To Workspace5/1, Controlled Voltage Source/1
  PS-Simulink Converter2/1 -> Controlled Voltage Source1/1
  PS-Simulink Converter3/1 -> Controlled Voltage Source6/1
  Demux11/1 -> Simulink-PS Converter12/1
  Demux11/2 -> Simulink-PS Converter13/1
  PS-Simulink Converter8/1 -> Controlled Voltage Source5/1
  [b1] -> Demux11/1
  [b3] -> Demux10/1
  PS-Simulink Converter7/1 -> Controlled Voltage Source4/1
  PS-Simulink Converter9/1 -> Controlled Voltage Source7/1
  PS-Simulink Converter5/1 -> Controlled Voltage Source3/1
  [c1] -> Demux12/1
  PS-Simulink Converter4/1 -> Controlled Voltage Source2/1
  PS-Simulink Converter6/1 -> Controlled Voltage Source8/1
  Voltage Measurement1/1 -> Scope/3, Simulink-PS Converter21/1
  Voltage Measurement4/1 -> Scope/2, Simulink-PS Converter20/1
  Voltage Measurement5/1 -> Scope/1, Simulink-PS Converter18/1
  Demux6/2 -> Simulink-PS Converter1/1
  [a9] -> Demux8/1
  Demux8/1 -> Simulink-PS Converter4/1
  Demux8/2 -> Simulink-PS Converter5/1
  [b9] -> Demux9/1
  Demux9/1 -> Simulink-PS Converter16/1
  Demux9/2 -> Simulink-PS Converter17/1
  Demux10/1 -> Simulink-PS Converter14/1
  Demux10/2 -> Simulink-PS Converter15/1
  Demux12/1 -> Simulink-PS Converter6/1
  Demux12/2 -> Simulink-PS Converter7/1
  [c3] -> Demux13/1
  Demux13/1 -> Simulink-PS Converter8/1
  Demux13/2 -> Simulink-PS Converter9/1
  [c9] -> Demux16/1
  Demux16/1 -> Simulink-PS Converter10/1
  Demux16/2 -> Simulink-PS Converter11/1
  PS-Simulink Converter12/1 -> Scope5/6
  PS-Simulink Converter11/1 -> Scope5/5
  PS-Simulink Converter10/1 -> To Workspace2/1, To Workspace4/1, Scope5/4
  Mux/1 -> MATLAB Function10/1(D)
  MATLAB Function10/1(Dout) -> Matrix Multiply/2
  Constant1/1 -> Matrix Multiply/1
  Matrix Multiply1/1 -> Demux17/1
  Constant/1 -> Matrix Multiply1/2
  Matrix Multiply/1 -> Matrix Multiply1/1
  MATLAB Function17/1(y) -> [b9]
  MATLAB Function19/1(y) -> [b1]
  MATLAB Function22/1(y) -> [c1]
  MATLAB Function16/1(y) -> [a1]
  Demux20/1 -> MATLAB Function14/1(u)  "a9"
  MATLAB Function15/1(y) -> [a3]
  MATLAB Function21/1(y) -> [c3]
  MATLAB Function18/1(y) -> [b3]
  Demux22/3 -> MATLAB Function22/1(u)  "c1"
  Demux22/2 -> MATLAB Function21/1(u)  "c3"
  Demux21/2 -> MATLAB Function18/1(u)  "b3"
  Demux21/1 -> MATLAB Function17/1(u)  "b9"
  MATLAB Function20/1(y) -> [c9]
  MATLAB Function11/1(ControlSignals) -> Demux21/1
  Demux20/3 -> MATLAB Function16/1(u)  "a1"
  MATLAB Function13/1(ControlSignals) -> Demux20/1  "a_cell_levels"
  Demux22/1 -> MATLAB Function20/1(u)  "c9"
  Demux21/3 -> MATLAB Function19/1(u)  "b1"
  Demux20/2 -> MATLAB Function15/1(u)  "a3"
  MATLAB Function12/1(ControlSignals) -> Demux22/1
  MATLAB Function14/1(y) -> [a9]
  MATLAB Function23/1(node_indices) -> Demux23/1
  Constant3/1 -> MATLAB Function23/5(n_levels)
  Constant2/1 -> MATLAB Function23/4(Vdc)
  Demux24/3 -> To Workspace12/1, MATLAB Function23/3(Ic)
  Demux24/2 -> MATLAB Function23/2(Ib)
  Demux23/1 -> To Workspace3/1, MATLAB Function13/1(V)
  Demux23/2 -> MATLAB Function11/1(V)
  Demux23/3 -> MATLAB Function12/1(V)
  Demux24/1 -> Scope6/1, To Workspace1/1, MATLAB Function23/1(Ia)
  PS-Simulink Converter13/1 -> To Workspace/1, Rate Transition2/1, Mux2/1, Scope3/4
  From2/1 -> Demux25/1
  Demux5/1 -> To Workspace9/1, Scope9/4
  Demux5/2 -> Scope9/5
  Demux5/3 -> Scope9/6
  Gain3/1 -> Goto1/1
  [ll_abc_reference] -> Demux5/1
  PS-Simulink Converter17/1 -> Scope9/2
  PS-Simulink Converter16/1 -> To Workspace11/1, Scope9/1
  PS-Simulink Converter18/1 -> Scope9/3
  THD/1 -> Scope13/1
  Demux26/3 -> Scope3/3  "ICc"
  [I_ll_sensed] -> Demux26/1
  Demux26/2 -> Scope3/2  "IBb"
  Demux26/1 -> Scope3/1  "IAa"
  Demux25/2 -> MATLAB Function24/2(Vb)
  Demux25/1 -> MATLAB Function24/1(Va)
  Demux25/3 -> MATLAB Function24/3(Vc)
  MATLAB Function24/1(Van) -> Sum2/2, Scope8/1, Sum/1, To Workspace7/1
  MATLAB Function24/3(Vcn) -> Sum2/1, Sum1/2, Scope8/3
  MATLAB Function24/2(Vbn) -> Sum/2, Sum1/1, Scope8/2
  Sum/1 -> Scope14/1
  Sum2/1 -> Scope14/3
  Sum1/1 -> Scope14/2
  PS-Simulink Converter19/1 -> Scope18/1, To Workspace10/1
  [ll_abc_reference] -> Demux27/1, Scope19/1
  Demux27/1 -> Data Type Conversion/1
  Data Type Conversion/1 -> Simulink-PS Converter19/1
  Rate Transition2/1 -> To Workspace6/1
  Rate Transition3/1 -> To Workspace13/1
  PS-Simulink Converter15/1 -> THD/1, Rate Transition3/1, Mux2/3, Scope3/6
  PS-Simulink Converter14/1 -> Mux2/2, Scope3/5
  Mux2/1 -> [I_meas]
  Gain6/1 -> Goto27/1
  Clock1/1 -> Gain6/1
  From21/1 -> abc to dq0/2
  ? -> abc to dq0/1
  From20/1 -> abc to dq1/1
  From22/1 -> abc to dq1/2
  abc to dq1/1 -> Sum3/2
  abc to dq0/1 -> Sum3/1
  Demux18/3 -> Discrete PID Controller2/1
  From23/1 -> dq0 to abc1/2
  Demux18/1 -> Discrete PID Controller/1
  Demux19/3 -> Scope20/3
  Sum3/1 -> Demux19/1, Demux18/1
  Demux19/1 -> Scope20/1
  Demux19/2 -> Scope20/2
  Discrete PID Controller1/1 -> Mux4/2
  Demux18/2 -> Discrete PID Controller1/1
  Mux4/1 -> Scope7/1, dq0 to abc1/1  "Controller output"
  Discrete PID Controller2/1 -> Mux4/3
  Discrete PID Controller/1 -> Mux4/1
  Mux1/1 -> Gain5/1
  Sine Wave1/1 -> Mux1/1
  Sine Wave2/1 -> Mux1/2
  Sine Wave6/1 -> Mux1/3
  Gain5/1 -> Rate Transition1/1
  Rate Transition1/1 -> Demux24/1
  connections:
  Full-Bridge Converter2/LConn2 -- Full-Bridge Converter/LConn1
  Full-Bridge Converter6/LConn1 -- Full-Bridge Converter4/LConn2
  Full-Bridge Converter7/LConn1 -- Full-Bridge Converter6/LConn2
  Full-Bridge Converter/LConn2 -- Full-Bridge Converter7/LConn2 -- Ground/LConn1 -- Full-Bridge Converter8/LConn2
  Vdc/ (400V)8/RConn1 -- Full-Bridge Converter8/RConn1
  Full-Bridge Converter8/RConn2 -- Vdc/ (400V)8/LConn1
  Full-Bridge Converter1/RConn2 -- Vdc/ (400V)7/LConn1
  Full-Bridge Converter1/RConn1 -- Vdc/ (400V)7/RConn1
  Full-Bridge Converter5/RConn2 -- Vdc/ (400V)6/LConn1
  Full-Bridge Converter5/RConn1 -- Vdc/ (400V)6/RConn1
  Full-Bridge Converter4/RConn1 -- Vdc/ (400V)5/RConn1
  Full-Bridge Converter4/RConn2 -- Vdc/ (400V)5/LConn1
  Full-Bridge Converter2/RConn1 -- Vdc/ (400V)/RConn1
  Full-Bridge Converter2/RConn2 -- Vdc/ (400V)/LConn1
  Full-Bridge Converter/RConn1 -- Vdc/ (400V)2/RConn1
  Full-Bridge Converter/RConn2 -- Vdc/ (400V)2/LConn1
  Full-Bridge Converter7/RConn2 -- Vdc/ (400V)3/LConn1
  Full-Bridge Converter7/RConn1 -- Vdc/ (400V)3/RConn1
  Full-Bridge Converter8/LConn1 -- Full-Bridge Converter1/LConn2
  Full-Bridge Converter1/LConn1 -- Full-Bridge Converter5/LConn2
  Full-Bridge Converter5/LConn1 -- Three-Phase V-I Measurement/LConn3
  Full-Bridge Converter4/LConn1 -- Three-Phase V-I Measurement/LConn2
  Full-Bridge Converter6/RConn2 -- Vdc/ (400V)4/LConn1
  Full-Bridge Converter6/RConn1 -- Vdc/ (400V)4/RConn1
  1 ohm 5 mH1/LConn1 -- Voltage Measurement/LConn1 -- Three-Phase V-I Measurement/RConn1
  1 ohm 5 mH2/LConn1 -- Voltage Measurement2/LConn1 -- Three-Phase V-I Measurement/RConn2
  1 ohm 5 mH3/LConn1 -- Voltage Measurement3/LConn1 -- Three-Phase V-I Measurement/RConn3
  1 ohm 5 mH3/RConn1 -- Voltage Measurement3/LConn2 -- Voltage Measurement2/LConn2 -- 1 ohm 5 mH2/RConn1 -- Voltage Measurement/LConn2 -- 1 ohm 5 mH1/RConn1
  Full-Bridge Converter2/LConn1 -- Three-Phase V-I Measurement/LConn1
  N-Channel MOSFET3/RConn2 -- Half-Bridge Driver1/RConn4 -- Solver Configuration/RConn1 -- Electrical Reference/LConn1 -- Voltage Source/RConn1 -- Half-Bridge Driver/RConn4 -- N-Channel MOSFET/RConn2
  N-Channel MOSFET3/RConn1 -- Voltage Sensor/RConn2 -- Half-Bridge Driver1/RConn2 -- N-Channel MOSFET2/RConn2
  N-Channel MOSFET/RConn1 -- Half-Bridge Driver/RConn2 -- Voltage Sensor/LConn1 -- N-Channel MOSFET1/RConn2
  N-Channel MOSFET1/RConn1 -- Voltage Source/LConn1 -- N-Channel MOSFET2/RConn1
  N-Channel MOSFET/LConn1 -- Half-Bridge Driver/RConn3
  Half-Bridge Driver/RConn1 -- N-Channel MOSFET1/LConn1
  Half-Bridge Driver1/RConn3 -- N-Channel MOSFET3/LConn1
  Half-Bridge Driver1/RConn1 -- N-Channel MOSFET2/LConn1
  Simulink-PS Converter1/RConn1 -- Half-Bridge Driver1/LConn1
  Simulink-PS Converter/RConn1 -- Half-Bridge Driver/LConn1
  N-Channel MOSFET6/RConn2 -- Voltage Sensor1/RConn2 -- Half-Bridge Driver3/RConn2 -- N-Channel MOSFET7/RConn1
  Voltage Source1/RConn1 -- Electrical Reference1/LConn1 -- Solver Configuration1/RConn1 -- N-Channel MOSFET7/RConn2 -- Half-Bridge Driver3/RConn4 -- Half-Bridge Driver2/RConn4 -- N-Channel MOSFET4/RConn2
  Half-Bridge Driver2/RConn2 -- N-Channel MOSFET4/RConn1 -- Voltage Sensor1/LConn1 -- N-Channel MOSFET5/RConn2
  N-Channel MOSFET6/RConn1 -- Voltage Source1/LConn1 -- N-Channel MOSFET5/RConn1
  Half-Bridge Driver3/RConn3 -- N-Channel MOSFET7/LConn1
  Half-Bridge Driver3/RConn1 -- N-Channel MOSFET6/LConn1
  Half-Bridge Driver2/RConn1 -- N-Channel MOSFET5/LConn1
  N-Channel MOSFET4/LConn1 -- Half-Bridge Driver2/RConn3
  Simulink-PS Converter2/RConn1 -- Half-Bridge Driver2/LConn1
  Simulink-PS Converter3/RConn1 -- Half-Bridge Driver3/LConn1
  PS-Simulink Converter1/LConn1 -- Voltage Sensor/RConn1
  PS-Simulink Converter2/LConn1 -- Voltage Sensor1/RConn1
  Controlled Voltage Source1/RConn1 -- Controlled Voltage Source/LConn1
  N-Channel MOSFET9/RConn1 -- N-Channel MOSFET10/RConn1 -- Voltage Source2/LConn1
  Solver Configuration2/RConn1 -- N-Channel MOSFET11/RConn2 -- Half-Bridge Driver5/RConn4 -- Voltage Source2/RConn1 -- Electrical Reference2/LConn1 -- Half-Bridge Driver4/RConn4 -- N-Channel MOSFET8/RConn2
  N-Channel MOSFET9/RConn2 -- Voltage Sensor2/LConn1 -- Half-Bridge Driver4/RConn2 -- N-Channel MOSFET8/RConn1
  N-Channel MOSFET11/RConn1 -- N-Channel MOSFET10/RConn2 -- Voltage Sensor2/RConn2 -- Half-Bridge Driver5/RConn2
  Simulink-PS Converter5/RConn1 -- Half-Bridge Driver5/LConn1
  Simulink-PS Converter4/RConn1 -- Half-Bridge Driver4/LConn1
  Half-Bridge Driver5/RConn1 -- N-Channel MOSFET10/LConn1
  Half-Bridge Driver5/RConn3 -- N-Channel MOSFET11/LConn1
  PS-Simulink Converter3/LConn1 -- Voltage Sensor2/RConn1
  N-Channel MOSFET8/LConn1 -- Half-Bridge Driver4/RConn3
  Half-Bridge Driver4/RConn1 -- N-Channel MOSFET9/LConn1
  N-Channel MOSFET31/RConn1 -- N-Channel MOSFET32/RConn1 -- Voltage Source7/LConn1
  N-Channel MOSFET24/RConn2 -- Half-Bridge Driver12/RConn4 -- N-Channel MOSFET29/RConn2 -- Half-Bridge Driver13/RConn4 -- Solver Configuration6/RConn1 -- Electrical Reference6/LConn1 -- Voltage Source6/RConn1
  N-Channel MOSFET33/RConn1 -- N-Channel MOSFET32/RConn2 -- Voltage Sensor7/RConn2 -- Half-Bridge Driver15/RConn2
  N-Channel MOSFET30/RConn2 -- Half-Bridge Driver14/RConn4 -- Voltage Source7/RConn1 -- Electrical Reference7/LConn1 -- Solver Configuration7/RConn1 -- N-Channel MOSFET33/RConn2 -- Half-Bridge Driver15/RConn4
  Half-Bridge Driver12/RConn2 -- N-Channel MOSFET24/RConn1 -- Voltage Sensor6/LConn1 -- N-Channel MOSFET25/RConn2
  N-Channel MOSFET34/RConn1 -- Half-Bridge Driver16/RConn2 -- Voltage Sensor8/LConn1 -- N-Channel MOSFET35/RConn2
  N-Channel MOSFET28/RConn2 -- N-Channel MOSFET29/RConn1 -- Voltage Sensor6/RConn2 -- Half-Bridge Driver13/RConn2
  N-Channel MOSFET27/RConn1 -- N-Channel MOSFET26/RConn2 -- Voltage Sensor8/RConn2 -- Half-Bridge Driver17/RConn2
  Electrical Reference8/LConn1 -- Voltage Source8/RConn1 -- Half-Bridge Driver16/RConn4 -- N-Channel MOSFET34/RConn2 -- Solver Configuration8/RConn1 -- N-Channel MOSFET27/RConn2 -- Half-Bridge Driver17/RConn4
  N-Channel MOSFET28/RConn1 -- N-Channel MOSFET25/RConn1 -- Voltage Source6/LConn1
  N-Channel MOSFET35/RConn1 -- N-Channel MOSFET26/RConn1 -- Voltage Source8/LConn1
  N-Channel MOSFET30/RConn1 -- Half-Bridge Driver14/RConn2 -- Voltage Sensor7/LConn1 -- N-Channel MOSFET31/RConn2
  Half-Bridge Driver15/RConn3 -- N-Channel MOSFET33/LConn1
  Half-Bridge Driver13/RConn3 -- N-Channel MOSFET29/LConn1
  Simulink-PS Converter13/RConn1 -- Half-Bridge Driver13/LConn1
  Half-Bridge Driver17/RConn1 -- N-Channel MOSFET26/LConn1
  Simulink-PS Converter14/RConn1 -- Half-Bridge Driver14/LConn1
  N-Channel MOSFET30/LConn1 -- Half-Bridge Driver14/RConn3
  Half-Bridge Driver14/RConn1 -- N-Channel MOSFET31/LConn1
  N-Channel MOSFET24/LConn1 -- Half-Bridge Driver12/RConn3
  Half-Bridge Driver16/RConn1 -- N-Channel MOSFET35/LConn1
  PS-Simulink Converter9/LConn1 -- Voltage Sensor8/RConn1
  Simulink-PS Converter16/RConn1 -- Half-Bridge Driver16/LConn1
  Half-Bridge Driver15/RConn1 -- N-Channel MOSFET32/LConn1
  Half-Bridge Driver13/RConn1 -- N-Channel MOSFET28/LConn1
  PS-Simulink Converter8/LConn1 -- Voltage Sensor7/RConn1
  N-Channel MOSFET34/LConn1 -- Half-Bridge Driver16/RConn3
  Simulink-PS Converter15/RConn1 -- Half-Bridge Driver15/LConn1
  Controlled Voltage Source5/RConn1 -- Controlled Voltage Source4/LConn1
  Simulink-PS Converter17/RConn1 -- Half-Bridge Driver17/LConn1
  Simulink-PS Converter12/RConn1 -- Half-Bridge Driver12/LConn1
  PS-Simulink Converter7/LConn1 -- Voltage Sensor6/RConn1
  Half-Bridge Driver17/RConn3 -- N-Channel MOSFET27/LConn1
  Half-Bridge Driver12/RConn1 -- N-Channel MOSFET25/LConn1
  N-Channel MOSFET19/RConn1 -- N-Channel MOSFET20/RConn1 -- Voltage Source4/LConn1
  N-Channel MOSFET12/RConn2 -- Half-Bridge Driver6/RConn4 -- N-Channel MOSFET17/RConn2 -- Half-Bridge Driver7/RConn4 -- Solver Configuration3/RConn1 -- Electrical Reference3/LConn1 -- Voltage Source3/RConn1
  N-Channel MOSFET21/RConn1 -- N-Channel MOSFET20/RConn2 -- Voltage Sensor4/RConn2 -- Half-Bridge Driver9/RConn2
  N-Channel MOSFET18/RConn2 -- Half-Bridge Driver8/RConn4 -- Voltage Source4/RConn1 -- Electrical Reference4/LConn1 -- Solver Configuration4/RConn1 -- N-Channel MOSFET21/RConn2 -- Half-Bridge Driver9/RConn4
  Half-Bridge Driver6/RConn2 -- N-Channel MOSFET12/RConn1 -- Voltage Sensor3/LConn1 -- N-Channel MOSFET13/RConn2
  N-Channel MOSFET22/RConn1 -- Half-Bridge Driver10/RConn2 -- Voltage Sensor5/LConn1 -- N-Channel MOSFET23/RConn2
  N-Channel MOSFET16/RConn2 -- N-Channel MOSFET17/RConn1 -- Voltage Sensor3/RConn2 -- Half-Bridge Driver7/RConn2
  N-Channel MOSFET15/RConn1 -- N-Channel MOSFET14/RConn2 -- Voltage Sensor5/RConn2 -- Half-Bridge Driver11/RConn2
  Electrical Reference5/LConn1 -- Voltage Source5/RConn1 -- Half-Bridge Driver10/RConn4 -- N-Channel MOSFET22/RConn2 -- Solver Configuration5/RConn1 -- N-Channel MOSFET15/RConn2 -- Half-Bridge Driver11/RConn4
  N-Channel MOSFET16/RConn1 -- N-Channel MOSFET13/RConn1 -- Voltage Source3/LConn1
  N-Channel MOSFET23/RConn1 -- N-Channel MOSFET14/RConn1 -- Voltage Source5/LConn1
  N-Channel MOSFET18/RConn1 -- Half-Bridge Driver8/RConn2 -- Voltage Sensor4/LConn1 -- N-Channel MOSFET19/RConn2
  Half-Bridge Driver9/RConn3 -- N-Channel MOSFET21/LConn1
  Half-Bridge Driver7/RConn3 -- N-Channel MOSFET17/LConn1
  Simulink-PS Converter7/RConn1 -- Half-Bridge Driver7/LConn1
  Half-Bridge Driver11/RConn1 -- N-Channel MOSFET14/LConn1
  Simulink-PS Converter8/RConn1 -- Half-Bridge Driver8/LConn1
  N-Channel MOSFET18/LConn1 -- Half-Bridge Driver8/RConn3
  Half-Bridge Driver8/RConn1 -- N-Channel MOSFET19/LConn1
  N-Channel MOSFET12/LConn1 -- Half-Bridge Driver6/RConn3
  Half-Bridge Driver10/RConn1 -- N-Channel MOSFET23/LConn1
  PS-Simulink Converter6/LConn1 -- Voltage Sensor5/RConn1
  Simulink-PS Converter10/RConn1 -- Half-Bridge Driver10/LConn1
  Half-Bridge Driver9/RConn1 -- N-Channel MOSFET20/LConn1
  Half-Bridge Driver7/RConn1 -- N-Channel MOSFET16/LConn1
  PS-Simulink Converter5/LConn1 -- Voltage Sensor4/RConn1
  N-Channel MOSFET22/LConn1 -- Half-Bridge Driver10/RConn3
  Simulink-PS Converter9/RConn1 -- Half-Bridge Driver9/LConn1
  Controlled Voltage Source3/RConn1 -- Controlled Voltage Source2/LConn1
  Simulink-PS Converter11/RConn1 -- Half-Bridge Driver11/LConn1
  Simulink-PS Converter6/RConn1 -- Half-Bridge Driver6/LConn1
  PS-Simulink Converter4/LConn1 -- Voltage Sensor3/RConn1
  Half-Bridge Driver11/RConn3 -- N-Channel MOSFET15/LConn1
  Half-Bridge Driver6/RConn1 -- N-Channel MOSFET13/LConn1
  Controlled Voltage Source6/RConn1 -- Controlled Voltage Source1/LConn1
  Controlled Voltage Source5/LConn1 -- Controlled Voltage Source7/RConn1
  Controlled Voltage Source8/RConn1 -- Controlled Voltage Source3/LConn1
  Ground1/LConn1 -- Controlled Voltage Source8/LConn1 -- Controlled Voltage Source6/LConn1 -- Controlled Voltage Source7/LConn1
  Simulink-PS Converter21/RConn1 -- Controlled Voltage Source11/RConn1
  Ground2/LConn1 -- Voltage Measurement1/LConn2
  Controlled Voltage Source2/RConn1 -- Voltage Measurement1/LConn1
  Voltage Sensor11/LConn1 -- Voltage Sensor13/RConn2 -- Inductor2/LConn1 -- Controlled Voltage Source11/LConn1 -- Voltage Sensor14/LConn1
  Controlled Voltage Source4/RConn1 -- Voltage Measurement4/LConn1
  Ground3/LConn1 -- Voltage Measurement4/LConn2
  Controlled Voltage Source/RConn1 -- Voltage Measurement5/LConn1
  Ground4/LConn1 -- Voltage Measurement5/LConn2
  Controlled Voltage Source9/RConn1 -- Simulink-PS Converter18/RConn1
  Controlled Voltage Source10/RConn1 -- Simulink-PS Converter20/RConn1
  Voltage Sensor14/RConn2 -- Voltage Sensor12/LConn1 -- Voltage Sensor9/LConn1 -- Inductor/LConn1 -- Controlled Voltage Source9/LConn1
  Controlled Voltage Source10/RConn2 -- Electrical Reference9/LConn1 -- Controlled Voltage Source9/RConn2 -- Solver Configuration9/RConn1 -- Controlled Voltage Source11/RConn2
  Voltage Sensor11/RConn2 -- Current Sensor2/RConn2 -- Current Sensor1/RConn2 -- Current Sensor/RConn2 -- Voltage Sensor9/RConn2 -- Voltage Sensor10/RConn2
  PS-Simulink Converter11/LConn1 -- Voltage Sensor10/RConn1
  PS-Simulink Converter10/LConn1 -- Voltage Sensor9/RConn1
  Voltage Sensor11/RConn1 -- PS-Simulink Converter12/LConn1
  Current Sensor/RConn1 -- PS-Simulink Converter13/LConn1
  Resistor2/RConn1 -- Current Sensor1/LConn1
  PS-Simulink Converter14/LConn1 -- Current Sensor1/RConn1
  Current Sensor2/LConn1 -- Resistor/RConn1
  Current Sensor2/RConn1 -- PS-Simulink Converter15/LConn1
  Current Sensor/LConn1 -- Resistor1/RConn1
  PS-Simulink Converter16/LConn1 -- Voltage Sensor12/RConn1
  PS-Simulink Converter17/LConn1 -- Voltage Sensor13/RConn1
  PS-Simulink Converter18/LConn1 -- Voltage Sensor14/RConn1
  Voltage Sensor10/LConn1 -- Inductor1/LConn1 -- Voltage Sensor13/LConn1 -- Controlled Voltage Source10/LConn1 -- Voltage Sensor12/RConn2
  Controlled Voltage Source12/RConn1 -- Simulink-PS Converter19/RConn1
  Electrical Reference10/LConn1 -- Solver Configuration10/RConn1 -- Controlled Voltage Source12/RConn2 -- Voltage Sensor15/RConn2
  PS-Simulink Converter19/LConn1 -- Voltage Sensor15/RConn1
  Controlled Voltage Source12/LConn1 -- Voltage Sensor15/LConn1
  Inductor/RConn1 -- Resistor1/LConn1
  Inductor1/RConn1 -- Resistor2/LConn1
  Inductor2/RConn1 -- Resistor/LConn1
